simulink model "ScriptDemo"  (R2022b)
settings: configuration reference "TmVcThermal_Configuration_sub" (kept outside this file)
undefined symbols (not defined in the file or in its folder): aaaa, bbbb, cTmComprCtrl_D_u8HvacFlowTable_db, cTmComprCtrl_D_u8HvacFlowTable_sw, cTmComprCtrl_n_i16ChillCmpIMax, cTmComprCtrl_n_i16ChillCmpIMin, cTmComprCtrl_n_i16ChillCmpIMin666, cTmComprCtrl_n_i16ChillCmpPMax, cTmComprCtrl_n_i16ChillCmpPMin, cTmComprCtrl_n_i16CmpChillCoolRpmKiMax, cTmComprCtrl_n_i16CmpChillCoolRpmKiMin, cTmComprCtrl_n_i16CmpChillCoolRpmKpMax, cTmComprCtrl_n_i16CmpChillCoolRpmKpMin, cTmComprCtrl_n_i16CmpCoolRpmKiMax, cTmComprCtrl_n_i16CmpCoolRpmKiMin, cTmComprCtrl_n_i16CmpCoolRpmKpMax, cTmComprCtrl_n_i16CmpCoolRpmKpMin, cTmComprCtrl_n_i16SM4CmpHeatKiMax, cTmComprCtrl_n_i16SM4CmpHeatKiMin, cTmComprCtrl_n_i16SM4CmpHeatKpMax, cTmComprCtrl_n_i16SM4CmpHeatKpMin, cTmComprCtrl_n_i16SM5CmpHeatKiMax, cTmComprCtrl_n_i16SM5CmpHeatKiMin, cTmComprCtrl_n_i16SM5CmpHeatKpMax, cTmComprCtrl_n_i16SM5CmpHeatKpMin, cTmComprCtrl_n_i16SM6CmpHeatKiMax, cTmComprCtrl_n_i16SM6CmpHeatKiMin, cTmComprCtrl_n_i16SM6CmpHeatKpMax, cTmComprCtrl_n_i16SM6CmpHeatKpMin, cTmComprCtrl_n_u16CmpMaxSpdFanFltLimt, cTmComprCtrl_n_u16CmpMaxSpdLoSidePFltLimt, cTmComprCtrl_n_u16CmpMaxSpdSensorFltLimt, cTmComprCtrl_n_u16CompMinRpm, cTmComprCtrl_n_u16CompRpmIncThres, cTmComprCtrl_t_u16BattCooltFFPeriod, cTmComprCtrl_t_u16BattCooltPIPeriod, cTmComprCtrl_t_u16CmpCoolFFPeriod, cTmComprCtrl_t_u16CmpCoolPIPeriod, cTmComprCtrl_t_u16CoolCmpChillFFPeriod, cTmComprCtrl_t_u16CoolCmpChillPIPeriod, cTmComprCtrl_t_u16SM4CmpHeatFFPeriod, cTmComprCtrl_t_u16SM4CmpHeatPIPeriod, cTmComprCtrl_t_u16SM5CmpHeatFFPeriod, cTmComprCtrl_t_u16SM5CmpHeatPIPeriod, cTmComprCtrl_t_u16SM6CmpHeatFFPeriod, cTmComprCtrl_t_u16SM6CmpHeatPIPeriod, cTmComprCtrl_Te_EvapClearInteg, cTmComprCtrl_Te_i16HpReqTempSaturoffset, cTmComprCtrl_Te_i16SatLpReplaceDiff, cTmComprCtrl_Te_i16SM3BatDiffStartEvapDecOffset, cTmComprCtrl_Te_i16SM3EvapLo, cTmComprCtrl_Te_i16SM3TBatDiffEntEvapDecOffset, cTmComprCtrl_Te_i16SM3TBatDiffEntEvapDecOffsetQuit, cTmComprCtrl_Te_s32ErrCmpChillPIContinueCoolH, cTmComprCtrl_Te_s32ErrCmpChillPIContinueCoolL, cTmComprCtrl_Te_s32ErrCmpPIContinueChillH, cTmComprCtrl_Te_s32ErrCmpPIContinueChillL, cTmComprCtrl_Te_s32ErrCmpPIContinueCoolH, cTmComprCtrl_Te_s32ErrCmpPIContinueCoolL, cTmComprCtrl_Te_s32ErrCmpPIContinueHeatH ... (+398)
libraries: simulink x846, PCMULib x711, simulink_need_slupdate x4
(part 14 of 49)

== system ScriptDemo/Change/changeModSizeGcs/Before1/Subsystem3 ==
  rTmComprCtrl_n_u16CompRpmReqModeOut : Inport  OutDataTypeStr=uint16
  sTmDiag_D_u8CmprDischrgTFltSt : Inport  Port=2  OutDataTypeStr=uint8
  sTmDiag_D_u8FanFltSt : Inport  Port=3  OutDataTypeStr=uint8
  sTmDiag_D_u8HiSidePFltSt : Inport  Port=4  OutDataTypeStr=uint8
  sTmDiag_D_u8OutrCondOutTFltSt : Inport  Port=5  OutDataTypeStr=uint8
  sTmIn_n_s32ElacCmprActl : Inport  Port=6  OutDataTypeStr=single
  sTmIn_v_s32VehSpdLgt : Inport  Port=7  OutDataTypeStr=single
  sTmRefriModeMgr_D_u8HpFmCmd : Inport  Port=8  OutDataTypeStr=uint8
  sTmSigProces_Pw_i16ReqPwrForHeat : Inport  Port=9  OutDataTypeStr=int16
  sTmSigProces_Te_s32CompDischarge : Inport  Port=10  OutDataTypeStr=single
  sTmSigProces_md_u16BlwCool : Inport  Port=11  OutDataTypeStr=uint16
  sTmSigProces_p_u16PHighSide : Inport  Port=12  OutDataTypeStr=uint16
  sTmSigProces_p_u16PLowSide : Inport  Port=13  OutDataTypeStr=uint16
  sTmIn_D_u8HeatPump : Inport  Port=14  OutDataTypeStr=uint8
  sTmIn_D_u8ElecDriveline : Inport  Port=15
  sTmSigProces_md_u16BlwHeat : Inport  Port=16  OutDataTypeStr=uint16
  sTmDiag_D_u8LoSidePFltSt : Inport  Port=17  OutDataTypeStr=uint8
  xTmComprCtrl_B_CompOnReqCompOn : Inport  Port=18  OutDataTypeStr=boolean
  rTmComprCtrl_n_u16CompRpmReqFilter : Outport  OutDataTypeStr=uint16
  xTmComprCtrl_B_KeepRpm : Outport  Port=2  OutDataTypeStr=boolean
  xFilter_B_ComprStop : Outport  Port=3  OutDataTypeStr=boolean
  sFilter_n_u16CompMaxRpm : Outport  Port=4  OutDataTypeStr=uint16
  rFilter_p_u16AcHiSideHiCut : Outport  Port=5  OutDataTypeStr=uint16
  rFilter_p_u16CmpLimitNormalP : Outport  Port=6  OutDataTypeStr=uint16
  rFilter_p_u16CmpLimitLowP : Outport  Port=7  OutDataTypeStr=uint16
  rFilter_p_u16CmpLimitMidP : Outport  Port=8  OutDataTypeStr=uint16
  rFilter_p_u16CmpLimitShutDownP : Outport  Port=9  OutDataTypeStr=uint16
  xTmComprCtrl_B_ReduceRpm : Outport  Port=10  OutDataTypeStr=boolean
  wires:
  ? -> [sTmRefriModeMgr_D_u8HPCurMode]
  sTmIn_n_s32ElacCmprActl/1 -> [sTmIn_n_s32ElacCmprActl]
  [rTmComprCtrl_p_u16AcHiSideHiCut] -> rFilter_p_u16AcHiSideHiCut/1
  sTmIn_D_u8HeatPump/1 -> [sTmIn_D_u8HeatPump]
  sTmSigProces_md_u16BlwCool/1 -> [sTmSigProces_md_u16BlwCool]
  sTmDiag_D_u8OutrCondOutTFltSt/1 -> [sTmDiag_D_u8OutrCondOutTFltSt]
  ? -> [sTmSigProces_Te_s32TAmb]
  sTmSigProces_md_u16BlwHeat/1 -> [sTmSigProces_md_u16BlwHeat]
  [rTmComprCtrl_p_u16CmpLimitShutDownP] -> rFilter_p_u16CmpLimitShutDownP/1
  sTmRefriModeMgr_D_u8HpFmCmd/1 -> [sTmRefriModeMgr_D_u8HpFmCmd]
  [rTmComprCtrl_p_u16CmpLimitLowP] -> rFilter_p_u16CmpLimitLowP/1
  sTmDiag_D_u8LoSidePFltSt/1 -> [sTmDiag_D_u8LoSidePFltSt]
  sTmSigProces_p_u16PLowSide/1 -> [sTmSigProces_p_u16PLowSide]
  [rTmComprCtrl_n_u16CompRpmReqCompOn] -> rTmComprCtrl_n_u16CompRpmReqFilter/1
  [xTmComprCtrl_B_ComprStop] -> xFilter_B_ComprStop/1
  sTmIn_D_u8ElecDriveline/1 -> [sTmIn_D_u8ElecDriveline]
  sTmDiag_D_u8HiSidePFltSt/1 -> [sTmDiag_D_u8HiSidePFltSt]
  [sTmComprCtrl_n_u16CompMaxRpm] -> sFilter_n_u16CompMaxRpm/1
  ? -> [sTmSigProces_D_u8CarChrgMode]
  [xTmComprCtrl_B_KeepRpm] -> xTmComprCtrl_B_KeepRpm/1
  sTmDiag_D_u8CmprDischrgTFltSt/1 -> [sTmDiag_D_u8CmprDischrgTFltSt]
  sTmSigProces_p_u16PHighSide/1 -> [sTmSigProces_p_u16PHighSide]
  xTmComprCtrl_B_CompOnReqCompOn/1 -> [xTmComprCtrl_B_CompOnReqCompOn]
  sTmSigProces_Te_s32CompDischarge/1 -> [sTmSigProces_Te_s32CompDischarge]
  [rTmComprCtrl_p_u16CmpLimitMidP] -> rFilter_p_u16CmpLimitMidP/1
  [rTmComprCtrl_p_u16CmpLimitNormalP] -> rFilter_p_u16CmpLimitNormalP/1
  sTmIn_v_s32VehSpdLgt/1 -> [sTmIn_v_s32VehSpdLgt]
  [xTmComprCtrl_B_ReduceRpm] -> xTmComprCtrl_B_ReduceRpm/1
  sTmSigProces_Pw_i16ReqPwrForHeat/1 -> [sTmSigProces_Pw_i16ReqPwrForHeat]
  sTmDiag_D_u8FanFltSt/1 -> [sTmDiag_D_u8FanFltSt]
  rTmComprCtrl_n_u16CompRpmReqModeOut/1 -> [rTmComprCtrl_n_u16CompRpmReqModeOut]

== system ScriptDemo/Create/Model/createModGoto/After ==
  note: % 目的: 为输出端口创建debug 及对应的输入模块
      | [cnt] = createDebug(gcs)
  note: <模型信息: After>
      |
      | 【输入端口】
      | sTmRefriVlvCtrl_X_s32CEXVPosReqIn
      | sTmRefriVlvCtrl_X_s32EEXVPosReqIn
      | sTmRefriVlvCtrl_X_s32BEXVPosReqIn
      | yTmRefriVlvCtrl_B_HpcCexvMovEnableIn
      | sTmRefriVlvCtrl_Z_u8CEXVInitStateIn
      | yTmRefriVlvCtrl_B_CexvCalibReqIn
      | yTmRefriVlvCtrl_B_HpcEexvMovEnableIn
      | sTmRefriVlvCtrl_Z_u8EEXVInitStateIn
      | yTmRefriVlvCtrl_B_EexvCalibReqIn
      | yTmRefriVlvCtrl_B_HpcBexvMovEnableIn
      | sTmRefriVlvCtrl_Z_u8BEXVInitStateIn
      | yTmRefriVlvCtrl_B_BexvCalibReqIn
      | sTmRefriVlvCtrl_X_s32SM3BexvMaxPosIn
      | yTmRefriVlvCtrl_B_EvapBattTLimBexvEnaIn
      | sTmRefriVlvCtrl_D_u8EexvRefriSwitchStIn
      | sTmRefriVlvCtrl_D_u8CexvRefriSwitchStIn
      | sTmRefriVlvCtrl_D_u8BexvRefriSwitchStIn
      |
      | 【输出端口】
      | sTmRefriVlvCtrl_X_s32CEXVPosReq
      | sTmRefriVlvCtrl_X_s32EEXVPosReq
      | sTmRefriVlvCtrl_X_s32BEXVPosReq
      | yTmRefriVlvCtrl_B_HpcCexvMovEnable
      | sTmRefriVlvCtrl_Z_u8CEXVInitState
      | yTmRefriVlvCtrl_B_CexvCalibReq
      | yTmRefriVlvCtrl_B_HpcEexvMovEnable
      | sTmRefriVlvCtrl_Z_u8EEXVInitState
      | yTmRefriVlvCtrl_B_EexvCalibReq
      | yTmRefriVlvCtrl_B_HpcBexvMovEnable
      | sTmRefriVlvCtrl_Z_u8BEXVInitState
      | yTmRefriVlvCtrl_B_BexvCalibReq
      | sTmRefriVlvCtrl_X_s32SM3BexvMaxPos
      | yTmRefriVlvCtrl_B_EvapBattTLimBexvEna
      | sTmRefriVlvCtrl_D_u8EexvRefriSwitchSt
      | sTmRefriVlvCtrl_D_u8CexvRefriSwitchSt
      | sTmRefriVlvCtrl_D_u8BexvRefriSwitchSt
      |
      | 【标定量】
      | 无标定量
      |
      | 创建时间: 2025-03-13 10:33:23
  sTmRefriVlvCtrl_X_s32CEXVPosReqIn : Inport  OutDataTypeStr=single
  sTmRefriVlvCtrl_X_s32EEXVPosReqIn : Inport  Port=2  OutDataTypeStr=single
  sTmRefriVlvCtrl_X_s32BEXVPosReqIn : Inport  Port=3  OutDataTypeStr=single
  yTmRefriVlvCtrl_B_HpcCexvMovEnableIn : Inport  Port=4  OutDataTypeStr=boolean
  sTmRefriVlvCtrl_Z_u8CEXVInitStateIn : Inport  Port=5  OutDataTypeStr=uint8
  yTmRefriVlvCtrl_B_CexvCalibReqIn : Inport  Port=6  OutDataTypeStr=boolean
  yTmRefriVlvCtrl_B_HpcEexvMovEnableIn : Inport  Port=7  OutDataTypeStr=boolean
  sTmRefriVlvCtrl_Z_u8EEXVInitStateIn : Inport  Port=8  OutDataTypeStr=uint8
  yTmRefriVlvCtrl_B_EexvCalibReqIn : Inport  Port=9  OutDataTypeStr=boolean
  yTmRefriVlvCtrl_B_HpcBexvMovEnableIn : Inport  Port=10  OutDataTypeStr=boolean
  sTmRefriVlvCtrl_Z_u8BEXVInitStateIn : Inport  Port=11  OutDataTypeStr=uint8
  yTmRefriVlvCtrl_B_BexvCalibReqIn : Inport  Port=12  OutDataTypeStr=boolean
  sTmRefriVlvCtrl_X_s32SM3BexvMaxPosIn : Inport  Port=13  OutDataTypeStr=single
  yTmRefriVlvCtrl_B_EvapBattTLimBexvEnaIn : Inport  Port=14  OutDataTypeStr=boolean
  sTmRefriVlvCtrl_D_u8EexvRefriSwitchStIn : Inport  Port=15  OutDataTypeStr=uint8
  sTmRefriVlvCtrl_D_u8CexvRefriSwitchStIn : Inport  Port=16  OutDataTypeStr=uint8
  sTmRefriVlvCtrl_D_u8BexvRefriSwitchStIn : Inport  Port=17  OutDataTypeStr=uint8
  OutDebug : PCMULib/Interface/OutdebugRvs  SWI=cTmRefriVlvCtrl_X_s32CEXVPosReq_sw  DBI=cTmRefriVlvCtrl_X_s32CEXVPosReq_db
      settings: SourceProductName=PCMULib
  OutDebug1 : PCMULib/Interface/OutdebugRvs  SWI=cTmRefriVlvCtrl_X_s32EEXVPosReq_sw  DBI=cTmRefriVlvCtrl_X_s32EEXVPosReq_db
      settings: SourceProductName=PCMULib
  OutDebug10 : PCMULib/Interface/OutdebugRvs  SWI=cTmRefriVlvCtrl_Z_u8BEXVInitState_sw  DBI=cTmRefriVlvCtrl_Z_u8BEXVInitState_db
      settings: SourceProductName=PCMULib
  OutDebug11 : PCMULib/Interface/OutdebugRvs  SWI=cTmRefriVlvCtrl_B_BexvCalibReq_sw  DBI=cTmRefriVlvCtrl_B_BexvCalibReq_db
      settings: SourceProductName=PCMULib
  OutDebug12 : PCMULib/Interface/OutdebugRvs  SWI=cTmRefriVlvCtrl_X_s32SM3BexvMaxPos_sw  DBI=cTmRefriVlvCtrl_X_s32SM3BexvMaxPos_db
      settings: SourceProductName=PCMULib
  OutDebug13 : PCMULib/Interface/OutdebugRvs  SWI=cTmRefriVlvCtrl_B_EvapBattTLimBexvEna_sw  DBI=cTmRefriVlvCtrl_B_EvapBattTLimBexvEna_db
      settings: SourceProductName=PCMULib
  OutDebug14 : PCMULib/Interface/OutdebugRvs  SWI=cTmRefriVlvCtrl_D_u8EexvRefriSwitchSt_sw  DBI=cTmRefriVlvCtrl_D_u8EexvRefriSwitchSt_db
      settings: SourceProductName=PCMULib
  OutDebug15 : PCMULib/Interface/OutdebugRvs  SWI=cTmRefriVlvCtrl_D_u8CexvRefriSwitchSt_sw  DBI=cTmRefriVlvCtrl_D_u8CexvRefriSwitchSt_db
      settings: SourceProductName=PCMULib
  OutDebug16 : PCMULib/Interface/OutdebugRvs  SWI=cTmRefriVlvCtrl_D_u8BexvRefriSwitchSt_sw  DBI=cTmRefriVlvCtrl_D_u8BexvRefriSwitchSt_db
      settings: SourceProductName=PCMULib
  OutDebug2 : PCMULib/Interface/OutdebugRvs  SWI=cTmRefriVlvCtrl_X_s32BEXVPosReq_sw  DBI=cTmRefriVlvCtrl_X_s32BEXVPosReq_db
      settings: SourceProductName=PCMULib
  OutDebug3 : PCMULib/Interface/OutdebugRvs  SWI=cTmRefriVlvCtrl_B_HpcCexvMovEnable_sw  DBI=cTmRefriVlvCtrl_B_HpcCexvMovEnable_db
      settings: SourceProductName=PCMULib
  OutDebug4 : PCMULib/Interface/OutdebugRvs  SWI=cTmRefriVlvCtrl_Z_u8CEXVInitState_sw  DBI=cTmRefriVlvCtrl_Z_u8CEXVInitState_db
      settings: SourceProductName=PCMULib
  OutDebug5 : PCMULib/Interface/OutdebugRvs  SWI=cTmRefriVlvCtrl_B_CexvCalibReq_sw  DBI=cTmRefriVlvCtrl_B_CexvCalibReq_db
      settings: SourceProductName=PCMULib
  OutDebug6 : PCMULib/Interface/OutdebugRvs  SWI=cTmRefriVlvCtrl_B_HpcEexvMovEnable_sw  DBI=cTmRefriVlvCtrl_B_HpcEexvMovEnable_db
      settings: SourceProductName=PCMULib
  OutDebug7 : PCMULib/Interface/OutdebugRvs  SWI=cTmRefriVlvCtrl_Z_u8EEXVInitState_sw  DBI=cTmRefriVlvCtrl_Z_u8EEXVInitState_db
      settings: SourceProductName=PCMULib
  OutDebug8 : PCMULib/Interface/OutdebugRvs  SWI=cTmRefriVlvCtrl_B_EexvCalibReq_sw  DBI=cTmRefriVlvCtrl_B_EexvCalibReq_db
      settings: SourceProductName=PCMULib
  OutDebug9 : PCMULib/Interface/OutdebugRvs  SWI=cTmRefriVlvCtrl_B_HpcBexvMovEnable_sw  DBI=cTmRefriVlvCtrl_B_HpcBexvMovEnable_db
      settings: SourceProductName=PCMULib
  sTmRefriVlvCtrl_X_s32CEXVPosReq : Outport  OutDataTypeStr=single
  sTmRefriVlvCtrl_X_s32EEXVPosReq : Outport  Port=2  OutDataTypeStr=single
  sTmRefriVlvCtrl_X_s32BEXVPosReq : Outport  Port=3  OutDataTypeStr=single
  yTmRefriVlvCtrl_B_HpcCexvMovEnable : Outport  Port=4  OutDataTypeStr=boolean
  sTmRefriVlvCtrl_Z_u8CEXVInitState : Outport  Port=5  OutDataTypeStr=uint8
  yTmRefriVlvCtrl_B_CexvCalibReq : Outport  Port=6  OutDataTypeStr=boolean
  yTmRefriVlvCtrl_B_HpcEexvMovEnable : Outport  Port=7  OutDataTypeStr=boolean
  sTmRefriVlvCtrl_Z_u8EEXVInitState : Outport  Port=8  OutDataTypeStr=uint8
  yTmRefriVlvCtrl_B_EexvCalibReq : Outport  Port=9  OutDataTypeStr=boolean
  yTmRefriVlvCtrl_B_HpcBexvMovEnable : Outport  Port=10  OutDataTypeStr=boolean
  sTmRefriVlvCtrl_Z_u8BEXVInitState : Outport  Port=11  OutDataTypeStr=uint8
  yTmRefriVlvCtrl_B_BexvCalibReq : Outport  Port=12  OutDataTypeStr=boolean
  sTmRefriVlvCtrl_X_s32SM3BexvMaxPos : Outport  Port=13  OutDataTypeStr=single
  yTmRefriVlvCtrl_B_EvapBattTLimBexvEna : Outport  Port=14  OutDataTypeStr=boolean
  sTmRefriVlvCtrl_D_u8EexvRefriSwitchSt : Outport  Port=15  OutDataTypeStr=uint8
  sTmRefriVlvCtrl_D_u8CexvRefriSwitchSt : Outport  Port=16  OutDataTypeStr=uint8
  sTmRefriVlvCtrl_D_u8BexvRefriSwitchSt : Outport  Port=17  OutDataTypeStr=uint8
  wires:
  sTmRefriVlvCtrl_X_s32SM3BexvMaxPosIn/1 -> OutDebug12/1
  OutDebug12/1 -> sTmRefriVlvCtrl_X_s32SM3BexvMaxPos/1
  sTmRefriVlvCtrl_X_s32BEXVPosReqIn/1 -> OutDebug2/1
  OutDebug2/1 -> sTmRefriVlvCtrl_X_s32BEXVPosReq/1
  OutDebug16/1 -> sTmRefriVlvCtrl_D_u8BexvRefriSwitchSt/1
  sTmRefriVlvCtrl_D_u8EexvRefriSwitchStIn/1 -> OutDebug14/1
  OutDebug5/1 -> yTmRefriVlvCtrl_B_CexvCalibReq/1
  OutDebug3/1 -> yTmRefriVlvCtrl_B_HpcCexvMovEnable/1
  sTmRefriVlvCtrl_Z_u8CEXVInitStateIn/1 -> OutDebug4/1
  OutDebug4/1 -> sTmRefriVlvCtrl_Z_u8CEXVInitState/1
  sTmRefriVlvCtrl_D_u8BexvRefriSwitchStIn/1 -> OutDebug16/1
  OutDebug1/1 -> sTmRefriVlvCtrl_X_s32EEXVPosReq/1
  OutDebug14/1 -> sTmRefriVlvCtrl_D_u8EexvRefriSwitchSt/1
  yTmRefriVlvCtrl_B_CexvCalibReqIn/1 -> OutDebug5/1
  sTmRefriVlvCtrl_X_s32EEXVPosReqIn/1 -> OutDebug1/1
  yTmRefriVlvCtrl_B_HpcCexvMovEnableIn/1 -> OutDebug3/1
  yTmRefriVlvCtrl_B_EvapBattTLimBexvEnaIn/1 -> OutDebug13/1
  OutDebug13/1 -> yTmRefriVlvCtrl_B_EvapBattTLimBexvEna/1
  sTmRefriVlvCtrl_Z_u8BEXVInitStateIn/1 -> OutDebug10/1
  OutDebug10/1 -> sTmRefriVlvCtrl_Z_u8BEXVInitState/1
  sTmRefriVlvCtrl_D_u8CexvRefriSwitchStIn/1 -> OutDebug15/1
  OutDebug15/1 -> sTmRefriVlvCtrl_D_u8CexvRefriSwitchSt/1
  OutDebug/1 -> sTmRefriVlvCtrl_X_s32CEXVPosReq/1
  OutDebug7/1 -> sTmRefriVlvCtrl_Z_u8EEXVInitState/1
  OutDebug8/1 -> yTmRefriVlvCtrl_B_EexvCalibReq/1
  yTmRefriVlvCtrl_B_EexvCalibReqIn/1 -> OutDebug8/1
  sTmRefriVlvCtrl_X_s32CEXVPosReqIn/1 -> OutDebug/1
  OutDebug6/1 -> yTmRefriVlvCtrl_B_HpcEexvMovEnable/1
  yTmRefriVlvCtrl_B_HpcEexvMovEnableIn/1 -> OutDebug6/1
  sTmRefriVlvCtrl_Z_u8EEXVInitStateIn/1 -> OutDebug7/1
  yTmRefriVlvCtrl_B_HpcBexvMovEnableIn/1 -> OutDebug9/1
  OutDebug9/1 -> yTmRefriVlvCtrl_B_HpcBexvMovEnable/1
  yTmRefriVlvCtrl_B_BexvCalibReqIn/1 -> OutDebug11/1
  OutDebug11/1 -> yTmRefriVlvCtrl_B_BexvCalibReq/1

== system ScriptDemo/Create/Model/createModGoto/After1 ==
  note: % 目的: 为输出端口创建debug 及对应的输入模块
      | [cnt] = createDebug(gcs)
  sTmRefriVlvCtrl_X_s32CEXVPosReqIn : Inport  OutDataTypeStr=single
  sTmRefriVlvCtrl_X_s32EEXVPosReqIn : Inport  Port=2  OutDataTypeStr=single
  sTmRefriVlvCtrl_X_s32BEXVPosReqIn : Inport  Port=3  OutDataTypeStr=single
  yTmRefriVlvCtrl_B_HpcCexvMovEnableIn : Inport  Port=4  OutDataTypeStr=boolean
  sTmRefriVlvCtrl_Z_u8CEXVInitStateIn : Inport  Port=5  OutDataTypeStr=uint8
  yTmRefriVlvCtrl_B_CexvCalibReqIn : Inport  Port=6  OutDataTypeStr=boolean
  yTmRefriVlvCtrl_B_HpcEexvMovEnableIn : Inport  Port=7  OutDataTypeStr=boolean
  sTmRefriVlvCtrl_Z_u8EEXVInitStateIn : Inport  Port=8  OutDataTypeStr=uint8
  yTmRefriVlvCtrl_B_EexvCalibReqIn : Inport  Port=9  OutDataTypeStr=boolean
  yTmRefriVlvCtrl_B_HpcBexvMovEnableIn : Inport  Port=10  OutDataTypeStr=boolean
  sTmRefriVlvCtrl_Z_u8BEXVInitStateIn : Inport  Port=11  OutDataTypeStr=uint8
  yTmRefriVlvCtrl_B_BexvCalibReqIn : Inport  Port=12  OutDataTypeStr=boolean
  sTmRefriVlvCtrl_X_s32SM3BexvMaxPosIn : Inport  Port=13  OutDataTypeStr=single
  yTmRefriVlvCtrl_B_EvapBattTLimBexvEnaIn : Inport  Port=14  OutDataTypeStr=boolean
  sTmRefriVlvCtrl_D_u8EexvRefriSwitchStIn : Inport  Port=15  OutDataTypeStr=uint8
  sTmRefriVlvCtrl_D_u8CexvRefriSwitchStIn : Inport  Port=16  OutDataTypeStr=uint8
  sTmRefriVlvCtrl_D_u8BexvRefriSwitchStIn : Inport  Port=17  OutDataTypeStr=uint8
  OutDebug : PCMULib/Interface/OutdebugRvs  SWI=cTmRefriVlvCtrl_X_s32CEXVPosReq_sw  DBI=cTmRefriVlvCtrl_X_s32CEXVPosReq_db
      settings: SourceProductName=PCMULib
  OutDebug1 : PCMULib/Interface/OutdebugRvs  SWI=cTmRefriVlvCtrl_X_s32EEXVPosReq_sw  DBI=cTmRefriVlvCtrl_X_s32EEXVPosReq_db
      settings: SourceProductName=PCMULib
  OutDebug10 : PCMULib/Interface/OutdebugRvs  SWI=cTmRefriVlvCtrl_Z_u8BEXVInitState_sw  DBI=cTmRefriVlvCtrl_Z_u8BEXVInitState_db
      settings: SourceProductName=PCMULib
  OutDebug11 : PCMULib/Interface/OutdebugRvs  SWI=cTmRefriVlvCtrl_B_BexvCalibReq_sw  DBI=cTmRefriVlvCtrl_B_BexvCalibReq_db
      settings: SourceProductName=PCMULib
  OutDebug12 : PCMULib/Interface/OutdebugRvs  SWI=cTmRefriVlvCtrl_X_s32SM3BexvMaxPos_sw  DBI=cTmRefriVlvCtrl_X_s32SM3BexvMaxPos_db
      settings: SourceProductName=PCMULib
  OutDebug13 : PCMULib/Interface/OutdebugRvs  SWI=cTmRefriVlvCtrl_B_EvapBattTLimBexvEna_sw  DBI=cTmRefriVlvCtrl_B_EvapBattTLimBexvEna_db
      settings: SourceProductName=PCMULib
  OutDebug14 : PCMULib/Interface/OutdebugRvs  SWI=cTmRefriVlvCtrl_D_u8EexvRefriSwitchSt_sw  DBI=cTmRefriVlvCtrl_D_u8EexvRefriSwitchSt_db
      settings: SourceProductName=PCMULib
  OutDebug15 : PCMULib/Interface/OutdebugRvs  SWI=cTmRefriVlvCtrl_D_u8CexvRefriSwitchSt_sw  DBI=cTmRefriVlvCtrl_D_u8CexvRefriSwitchSt_db
      settings: SourceProductName=PCMULib
  OutDebug16 : PCMULib/Interface/OutdebugRvs  SWI=cTmRefriVlvCtrl_D_u8BexvRefriSwitchSt_sw  DBI=cTmRefriVlvCtrl_D_u8BexvRefriSwitchSt_db
      settings: SourceProductName=PCMULib
  OutDebug2 : PCMULib/Interface/OutdebugRvs  SWI=cTmRefriVlvCtrl_X_s32BEXVPosReq_sw  DBI=cTmRefriVlvCtrl_X_s32BEXVPosReq_db
      settings: SourceProductName=PCMULib
  OutDebug3 : PCMULib/Interface/OutdebugRvs  SWI=cTmRefriVlvCtrl_B_HpcCexvMovEnable_sw  DBI=cTmRefriVlvCtrl_B_HpcCexvMovEnable_db
      settings: SourceProductName=PCMULib
  OutDebug4 : PCMULib/Interface/OutdebugRvs  SWI=cTmRefriVlvCtrl_Z_u8CEXVInitState_sw  DBI=cTmRefriVlvCtrl_Z_u8CEXVInitState_db
      settings: SourceProductName=PCMULib
  OutDebug5 : PCMULib/Interface/OutdebugRvs  SWI=cTmRefriVlvCtrl_B_CexvCalibReq_sw  DBI=cTmRefriVlvCtrl_B_CexvCalibReq_db
      settings: SourceProductName=PCMULib
  OutDebug6 : PCMULib/Interface/OutdebugRvs  SWI=cTmRefriVlvCtrl_B_HpcEexvMovEnable_sw  DBI=cTmRefriVlvCtrl_B_HpcEexvMovEnable_db
      settings: SourceProductName=PCMULib
  OutDebug7 : PCMULib/Interface/OutdebugRvs  SWI=cTmRefriVlvCtrl_Z_u8EEXVInitState_sw  DBI=cTmRefriVlvCtrl_Z_u8EEXVInitState_db
      settings: SourceProductName=PCMULib
  OutDebug8 : PCMULib/Interface/OutdebugRvs  SWI=cTmRefriVlvCtrl_B_EexvCalibReq_sw  DBI=cTmRefriVlvCtrl_B_EexvCalibReq_db
      settings: SourceProductName=PCMULib
  OutDebug9 : PCMULib/Interface/OutdebugRvs  SWI=cTmRefriVlvCtrl_B_HpcBexvMovEnable_sw  DBI=cTmRefriVlvCtrl_B_HpcBexvMovEnable_db
      settings: SourceProductName=PCMULib
  sTmRefriVlvCtrl_X_s32CEXVPosReq : Outport  OutDataTypeStr=single
  sTmRefriVlvCtrl_X_s32EEXVPosReq : Outport  Port=2  OutDataTypeStr=single
  sTmRefriVlvCtrl_X_s32BEXVPosReq : Outport  Port=3  OutDataTypeStr=single
  yTmRefriVlvCtrl_B_HpcCexvMovEnable : Outport  Port=4  OutDataTypeStr=boolean
  sTmRefriVlvCtrl_Z_u8CEXVInitState : Outport  Port=5  OutDataTypeStr=uint8
  yTmRefriVlvCtrl_B_CexvCalibReq : Outport  Port=6  OutDataTypeStr=boolean
  yTmRefriVlvCtrl_B_HpcEexvMovEnable : Outport  Port=7  OutDataTypeStr=boolean
  sTmRefriVlvCtrl_Z_u8EEXVInitState : Outport  Port=8  OutDataTypeStr=uint8
  yTmRefriVlvCtrl_B_EexvCalibReq : Outport  Port=9  OutDataTypeStr=boolean
  yTmRefriVlvCtrl_B_HpcBexvMovEnable : Outport  Port=10  OutDataTypeStr=boolean
  sTmRefriVlvCtrl_Z_u8BEXVInitState : Outport  Port=11  OutDataTypeStr=uint8
  yTmRefriVlvCtrl_B_BexvCalibReq : Outport  Port=12  OutDataTypeStr=boolean
  sTmRefriVlvCtrl_X_s32SM3BexvMaxPos : Outport  Port=13  OutDataTypeStr=single
  yTmRefriVlvCtrl_B_EvapBattTLimBexvEna : Outport  Port=14  OutDataTypeStr=boolean
  sTmRefriVlvCtrl_D_u8EexvRefriSwitchSt : Outport  Port=15  OutDataTypeStr=uint8
  sTmRefriVlvCtrl_D_u8CexvRefriSwitchSt : Outport  Port=16  OutDataTypeStr=uint8
  sTmRefriVlvCtrl_D_u8BexvRefriSwitchSt : Outport  Port=17  OutDataTypeStr=uint8
  wires:
  sTmRefriVlvCtrl_X_s32SM3BexvMaxPosIn/1 -> OutDebug12/1
  OutDebug12/1 -> sTmRefriVlvCtrl_X_s32SM3BexvMaxPos/1
  sTmRefriVlvCtrl_X_s32BEXVPosReqIn/1 -> OutDebug2/1
  OutDebug2/1 -> sTmRefriVlvCtrl_X_s32BEXVPosReq/1
  OutDebug16/1 -> sTmRefriVlvCtrl_D_u8BexvRefriSwitchSt/1
  sTmRefriVlvCtrl_D_u8EexvRefriSwitchStIn/1 -> OutDebug14/1
  OutDebug5/1 -> yTmRefriVlvCtrl_B_CexvCalibReq/1
  OutDebug3/1 -> yTmRefriVlvCtrl_B_HpcCexvMovEnable/1
  sTmRefriVlvCtrl_Z_u8CEXVInitStateIn/1 -> OutDebug4/1
  OutDebug4/1 -> sTmRefriVlvCtrl_Z_u8CEXVInitState/1
  sTmRefriVlvCtrl_D_u8BexvRefriSwitchStIn/1 -> OutDebug16/1
  OutDebug1/1 -> sTmRefriVlvCtrl_X_s32EEXVPosReq/1
  OutDebug14/1 -> sTmRefriVlvCtrl_D_u8EexvRefriSwitchSt/1
  yTmRefriVlvCtrl_B_CexvCalibReqIn/1 -> OutDebug5/1
  sTmRefriVlvCtrl_X_s32EEXVPosReqIn/1 -> OutDebug1/1
  yTmRefriVlvCtrl_B_HpcCexvMovEnableIn/1 -> OutDebug3/1
  yTmRefriVlvCtrl_B_EvapBattTLimBexvEnaIn/1 -> OutDebug13/1
  OutDebug13/1 -> yTmRefriVlvCtrl_B_EvapBattTLimBexvEna/1
  sTmRefriVlvCtrl_Z_u8BEXVInitStateIn/1 -> OutDebug10/1
  OutDebug10/1 -> sTmRefriVlvCtrl_Z_u8BEXVInitState/1
  sTmRefriVlvCtrl_D_u8CexvRefriSwitchStIn/1 -> OutDebug15/1
  OutDebug15/1 -> sTmRefriVlvCtrl_D_u8CexvRefriSwitchSt/1
  OutDebug/1 -> sTmRefriVlvCtrl_X_s32CEXVPosReq/1
  OutDebug7/1 -> sTmRefriVlvCtrl_Z_u8EEXVInitState/1
  OutDebug8/1 -> yTmRefriVlvCtrl_B_EexvCalibReq/1
  yTmRefriVlvCtrl_B_EexvCalibReqIn/1 -> OutDebug8/1
  sTmRefriVlvCtrl_X_s32CEXVPosReqIn/1 -> OutDebug/1
  OutDebug6/1 -> yTmRefriVlvCtrl_B_HpcEexvMovEnable/1
  yTmRefriVlvCtrl_B_HpcEexvMovEnableIn/1 -> OutDebug6/1
  sTmRefriVlvCtrl_Z_u8EEXVInitStateIn/1 -> OutDebug7/1
  yTmRefriVlvCtrl_B_HpcBexvMovEnableIn/1 -> OutDebug9/1
  OutDebug9/1 -> yTmRefriVlvCtrl_B_HpcBexvMovEnable/1
  yTmRefriVlvCtrl_B_BexvCalibReqIn/1 -> OutDebug11/1
  OutDebug11/1 -> yTmRefriVlvCtrl_B_BexvCalibReq/1

== system ScriptDemo/Create/Model/createModGoto/After2 ==
  note: % 目的: 为输出端口创建debug 及对应的输入模块
      | [cnt] = createDebug(gcs)
  sTmRefriVlvCtrl_X_s32CEXVPosReqIn : Inport  OutDataTypeStr=single
  sTmRefriVlvCtrl_X_s32EEXVPosReqIn : Inport  Port=2  OutDataTypeStr=single
  sTmRefriVlvCtrl_X_s32BEXVPosReqIn : Inport  Port=3  OutDataTypeStr=single
  yTmRefriVlvCtrl_B_HpcCexvMovEnableIn : Inport  Port=4  OutDataTypeStr=boolean
  sTmRefriVlvCtrl_Z_u8CEXVInitStateIn : Inport  Port=5  OutDataTypeStr=uint8
  yTmRefriVlvCtrl_B_CexvCalibReqIn : Inport  Port=6  OutDataTypeStr=boolean
  yTmRefriVlvCtrl_B_HpcEexvMovEnableIn : Inport  Port=7  OutDataTypeStr=boolean
  sTmRefriVlvCtrl_Z_u8EEXVInitStateIn : Inport  Port=8  OutDataTypeStr=uint8
  yTmRefriVlvCtrl_B_EexvCalibReqIn : Inport  Port=9  OutDataTypeStr=boolean
  yTmRefriVlvCtrl_B_HpcBexvMovEnableIn : Inport  Port=10  OutDataTypeStr=boolean
  sTmRefriVlvCtrl_Z_u8BEXVInitStateIn : Inport  Port=11  OutDataTypeStr=uint8
  yTmRefriVlvCtrl_B_BexvCalibReqIn : Inport  Port=12  OutDataTypeStr=boolean
  sTmRefriVlvCtrl_X_s32SM3BexvMaxPosIn : Inport  Port=13  OutDataTypeStr=single
  yTmRefriVlvCtrl_B_EvapBattTLimBexvEnaIn : Inport  Port=14  OutDataTypeStr=boolean
  sTmRefriVlvCtrl_D_u8EexvRefriSwitchStIn : Inport  Port=15  OutDataTypeStr=uint8
  sTmRefriVlvCtrl_D_u8CexvRefriSwitchStIn : Inport  Port=16  OutDataTypeStr=uint8
  sTmRefriVlvCtrl_D_u8BexvRefriSwitchStIn : Inport  Port=17  OutDataTypeStr=uint8
  OutDebug : PCMULib/Interface/OutdebugRvs  SWI=cTmRefriVlvCtrl_X_s32CEXVPosReq_sw  DBI=cTmRefriVlvCtrl_X_s32CEXVPosReq_db
      settings: SourceProductName=PCMULib
  OutDebug1 : PCMULib/Interface/OutdebugRvs  SWI=cTmRefriVlvCtrl_X_s32EEXVPosReq_sw  DBI=cTmRefriVlvCtrl_X_s32EEXVPosReq_db
      settings: SourceProductName=PCMULib
  OutDebug10 : PCMULib/Interface/OutdebugRvs  SWI=cTmRefriVlvCtrl_Z_u8BEXVInitState_sw  DBI=cTmRefriVlvCtrl_Z_u8BEXVInitState_db
      settings: SourceProductName=PCMULib
  OutDebug11 : PCMULib/Interface/OutdebugRvs  SWI=cTmRefriVlvCtrl_B_BexvCalibReq_sw  DBI=cTmRefriVlvCtrl_B_BexvCalibReq_db
      settings: SourceProductName=PCMULib
  OutDebug12 : PCMULib/Interface/OutdebugRvs  SWI=cTmRefriVlvCtrl_X_s32SM3BexvMaxPos_sw  DBI=cTmRefriVlvCtrl_X_s32SM3BexvMaxPos_db
      settings: SourceProductName=PCMULib
  OutDebug13 : PCMULib/Interface/OutdebugRvs  SWI=cTmRefriVlvCtrl_B_EvapBattTLimBexvEna_sw  DBI=cTmRefriVlvCtrl_B_EvapBattTLimBexvEna_db
      settings: SourceProductName=PCMULib
  OutDebug14 : PCMULib/Interface/OutdebugRvs  SWI=cTmRefriVlvCtrl_D_u8EexvRefriSwitchSt_sw  DBI=cTmRefriVlvCtrl_D_u8EexvRefriSwitchSt_db
      settings: SourceProductName=PCMULib
  OutDebug15 : PCMULib/Interface/OutdebugRvs  SWI=cTmRefriVlvCtrl_D_u8CexvRefriSwitchSt_sw  DBI=cTmRefriVlvCtrl_D_u8CexvRefriSwitchSt_db
      settings: SourceProductName=PCMULib
  OutDebug16 : PCMULib/Interface/OutdebugRvs  SWI=cTmRefriVlvCtrl_D_u8BexvRefriSwitchSt_sw  DBI=cTmRefriVlvCtrl_D_u8BexvRefriSwitchSt_db
      settings: SourceProductName=PCMULib
  OutDebug2 : PCMULib/Interface/OutdebugRvs  SWI=cTmRefriVlvCtrl_X_s32BEXVPosReq_sw  DBI=cTmRefriVlvCtrl_X_s32BEXVPosReq_db
      settings: SourceProductName=PCMULib
  OutDebug3 : PCMULib/Interface/OutdebugRvs  SWI=cTmRefriVlvCtrl_B_HpcCexvMovEnable_sw  DBI=cTmRefriVlvCtrl_B_HpcCexvMovEnable_db
      settings: SourceProductName=PCMULib
  OutDebug4 : PCMULib/Interface/OutdebugRvs  SWI=cTmRefriVlvCtrl_Z_u8CEXVInitState_sw  DBI=cTmRefriVlvCtrl_Z_u8CEXVInitState_db
      settings: SourceProductName=PCMULib
  OutDebug5 : PCMULib/Interface/OutdebugRvs  SWI=cTmRefriVlvCtrl_B_CexvCalibReq_sw  DBI=cTmRefriVlvCtrl_B_CexvCalibReq_db
      settings: SourceProductName=PCMULib
  OutDebug6 : PCMULib/Interface/OutdebugRvs  SWI=cTmRefriVlvCtrl_B_HpcEexvMovEnable_sw  DBI=cTmRefriVlvCtrl_B_HpcEexvMovEnable_db
      settings: SourceProductName=PCMULib
  OutDebug7 : PCMULib/Interface/OutdebugRvs  SWI=cTmRefriVlvCtrl_Z_u8EEXVInitState_sw  DBI=cTmRefriVlvCtrl_Z_u8EEXVInitState_db
      settings: SourceProductName=PCMULib
  OutDebug8 : PCMULib/Interface/OutdebugRvs  SWI=cTmRefriVlvCtrl_B_EexvCalibReq_sw  DBI=cTmRefriVlvCtrl_B_EexvCalibReq_db
      settings: SourceProductName=PCMULib
  OutDebug9 : PCMULib/Interface/OutdebugRvs  SWI=cTmRefriVlvCtrl_B_HpcBexvMovEnable_sw  DBI=cTmRefriVlvCtrl_B_HpcBexvMovEnable_db
      settings: SourceProductName=PCMULib
  sTmRefriVlvCtrl_X_s32CEXVPosReq : Outport  OutDataTypeStr=single
  sTmRefriVlvCtrl_X_s32EEXVPosReq : Outport  Port=2  OutDataTypeStr=single
  sTmRefriVlvCtrl_X_s32BEXVPosReq : Outport  Port=3  OutDataTypeStr=single
  yTmRefriVlvCtrl_B_HpcCexvMovEnable : Outport  Port=4  OutDataTypeStr=boolean
  sTmRefriVlvCtrl_Z_u8CEXVInitState : Outport  Port=5  OutDataTypeStr=uint8
  yTmRefriVlvCtrl_B_CexvCalibReq : Outport  Port=6  OutDataTypeStr=boolean
  yTmRefriVlvCtrl_B_HpcEexvMovEnable : Outport  Port=7  OutDataTypeStr=boolean
  sTmRefriVlvCtrl_Z_u8EEXVInitState : Outport  Port=8  OutDataTypeStr=uint8
  yTmRefriVlvCtrl_B_EexvCalibReq : Outport  Port=9  OutDataTypeStr=boolean
  yTmRefriVlvCtrl_B_HpcBexvMovEnable : Outport  Port=10  OutDataTypeStr=boolean
  sTmRefriVlvCtrl_Z_u8BEXVInitState : Outport  Port=11  OutDataTypeStr=uint8
  yTmRefriVlvCtrl_B_BexvCalibReq : Outport  Port=12  OutDataTypeStr=boolean
  sTmRefriVlvCtrl_X_s32SM3BexvMaxPos : Outport  Port=13  OutDataTypeStr=single
  yTmRefriVlvCtrl_B_EvapBattTLimBexvEna : Outport  Port=14  OutDataTypeStr=boolean
  sTmRefriVlvCtrl_D_u8EexvRefriSwitchSt : Outport  Port=15  OutDataTypeStr=uint8
  sTmRefriVlvCtrl_D_u8CexvRefriSwitchSt : Outport  Port=16  OutDataTypeStr=uint8
  sTmRefriVlvCtrl_D_u8BexvRefriSwitchSt : Outport  Port=17  OutDataTypeStr=uint8
  wires:
  sTmRefriVlvCtrl_X_s32SM3BexvMaxPosIn/1 -> OutDebug12/1
  OutDebug12/1 -> sTmRefriVlvCtrl_X_s32SM3BexvMaxPos/1
  sTmRefriVlvCtrl_X_s32BEXVPosReqIn/1 -> OutDebug2/1
  OutDebug2/1 -> sTmRefriVlvCtrl_X_s32BEXVPosReq/1
  OutDebug16/1 -> sTmRefriVlvCtrl_D_u8BexvRefriSwitchSt/1
  sTmRefriVlvCtrl_D_u8EexvRefriSwitchStIn/1 -> OutDebug14/1
  OutDebug5/1 -> yTmRefriVlvCtrl_B_CexvCalibReq/1
  OutDebug3/1 -> yTmRefriVlvCtrl_B_HpcCexvMovEnable/1
  sTmRefriVlvCtrl_Z_u8CEXVInitStateIn/1 -> OutDebug4/1
  OutDebug4/1 -> sTmRefriVlvCtrl_Z_u8CEXVInitState/1
  sTmRefriVlvCtrl_D_u8BexvRefriSwitchStIn/1 -> OutDebug16/1
  OutDebug1/1 -> sTmRefriVlvCtrl_X_s32EEXVPosReq/1
  OutDebug14/1 -> sTmRefriVlvCtrl_D_u8EexvRefriSwitchSt/1
  yTmRefriVlvCtrl_B_CexvCalibReqIn/1 -> OutDebug5/1
  sTmRefriVlvCtrl_X_s32EEXVPosReqIn/1 -> OutDebug1/1
  yTmRefriVlvCtrl_B_HpcCexvMovEnableIn/1 -> OutDebug3/1
  yTmRefriVlvCtrl_B_EvapBattTLimBexvEnaIn/1 -> OutDebug13/1
  OutDebug13/1 -> yTmRefriVlvCtrl_B_EvapBattTLimBexvEna/1
  sTmRefriVlvCtrl_Z_u8BEXVInitStateIn/1 -> OutDebug10/1
  OutDebug10/1 -> sTmRefriVlvCtrl_Z_u8BEXVInitState/1
  sTmRefriVlvCtrl_D_u8CexvRefriSwitchStIn/1 -> OutDebug15/1
  OutDebug15/1 -> sTmRefriVlvCtrl_D_u8CexvRefriSwitchSt/1
  OutDebug/1 -> sTmRefriVlvCtrl_X_s32CEXVPosReq/1
  OutDebug7/1 -> sTmRefriVlvCtrl_Z_u8EEXVInitState/1
  OutDebug8/1 -> yTmRefriVlvCtrl_B_EexvCalibReq/1
  yTmRefriVlvCtrl_B_EexvCalibReqIn/1 -> OutDebug8/1
  sTmRefriVlvCtrl_X_s32CEXVPosReqIn/1 -> OutDebug/1
  OutDebug6/1 -> yTmRefriVlvCtrl_B_HpcEexvMovEnable/1
  yTmRefriVlvCtrl_B_HpcEexvMovEnableIn/1 -> OutDebug6/1
  sTmRefriVlvCtrl_Z_u8EEXVInitStateIn/1 -> OutDebug7/1
  yTmRefriVlvCtrl_B_HpcBexvMovEnableIn/1 -> OutDebug9/1
  OutDebug9/1 -> yTmRefriVlvCtrl_B_HpcBexvMovEnable/1
  yTmRefriVlvCtrl_B_BexvCalibReqIn/1 -> OutDebug11/1
  OutDebug11/1 -> yTmRefriVlvCtrl_B_BexvCalibReq/1

== system ScriptDemo/Create/Model/createModGoto/After3 ==
  note: % 目的: 为输出端口创建debug 及对应的输入模块
      | [cnt] = createDebug(gcs)
  sTmRefriVlvCtrl_X_s32CEXVPosReqIn : Inport  OutDataTypeStr=single
  sTmRefriVlvCtrl_X_s32EEXVPosReqIn : Inport  Port=2  OutDataTypeStr=single
  sTmRefriVlvCtrl_X_s32BEXVPosReqIn : Inport  Port=3  OutDataTypeStr=single
  yTmRefriVlvCtrl_B_HpcCexvMovEnableIn : Inport  Port=4  OutDataTypeStr=boolean
  sTmRefriVlvCtrl_Z_u8CEXVInitStateIn : Inport  Port=5  OutDataTypeStr=uint8
  yTmRefriVlvCtrl_B_CexvCalibReqIn : Inport  Port=6  OutDataTypeStr=boolean
  yTmRefriVlvCtrl_B_HpcEexvMovEnableIn : Inport  Port=7  OutDataTypeStr=boolean
  sTmRefriVlvCtrl_Z_u8EEXVInitStateIn : Inport  Port=8  OutDataTypeStr=uint8
  yTmRefriVlvCtrl_B_EexvCalibReqIn : Inport  Port=9  OutDataTypeStr=boolean
  yTmRefriVlvCtrl_B_HpcBexvMovEnableIn : Inport  Port=10  OutDataTypeStr=boolean
  sTmRefriVlvCtrl_Z_u8BEXVInitStateIn : Inport  Port=11  OutDataTypeStr=uint8
  yTmRefriVlvCtrl_B_BexvCalibReqIn : Inport  Port=12  OutDataTypeStr=boolean
  sTmRefriVlvCtrl_X_s32SM3BexvMaxPosIn : Inport  Port=13  OutDataTypeStr=single
  yTmRefriVlvCtrl_B_EvapBattTLimBexvEnaIn : Inport  Port=14  OutDataTypeStr=boolean
  sTmRefriVlvCtrl_D_u8EexvRefriSwitchStIn : Inport  Port=15  OutDataTypeStr=uint8
  sTmRefriVlvCtrl_D_u8CexvRefriSwitchStIn : Inport  Port=16  OutDataTypeStr=uint8
  sTmRefriVlvCtrl_D_u8BexvRefriSwitchStIn : Inport  Port=17  OutDataTypeStr=uint8
  OutDebug : PCMULib/Interface/OutdebugRvs  SWI=cTmRefriVlvCtrl_X_s32CEXVPosReq_sw  DBI=cTmRefriVlvCtrl_X_s32CEXVPosReq_db
      settings: SourceProductName=PCMULib
  OutDebug1 : PCMULib/Interface/OutdebugRvs  SWI=cTmRefriVlvCtrl_X_s32EEXVPosReq_sw  DBI=cTmRefriVlvCtrl_X_s32EEXVPosReq_db
      settings: SourceProductName=PCMULib
  OutDebug10 : PCMULib/Interface/OutdebugRvs  SWI=cTmRefriVlvCtrl_Z_u8BEXVInitState_sw  DBI=cTmRefriVlvCtrl_Z_u8BEXVInitState_db
      settings: SourceProductName=PCMULib
  OutDebug11 : PCMULib/Interface/OutdebugRvs  SWI=cTmRefriVlvCtrl_B_BexvCalibReq_sw  DBI=cTmRefriVlvCtrl_B_BexvCalibReq_db
      settings: SourceProductName=PCMULib
  OutDebug12 : PCMULib/Interface/OutdebugRvs  SWI=cTmRefriVlvCtrl_X_s32SM3BexvMaxPos_sw  DBI=cTmRefriVlvCtrl_X_s32SM3BexvMaxPos_db
      settings: SourceProductName=PCMULib
  OutDebug13 : PCMULib/Interface/OutdebugRvs  SWI=cTmRefriVlvCtrl_B_EvapBattTLimBexvEna_sw  DBI=cTmRefriVlvCtrl_B_EvapBattTLimBexvEna_db
      settings: SourceProductName=PCMULib
  OutDebug14 : PCMULib/Interface/OutdebugRvs  SWI=cTmRefriVlvCtrl_D_u8EexvRefriSwitchSt_sw  DBI=cTmRefriVlvCtrl_D_u8EexvRefriSwitchSt_db
      settings: SourceProductName=PCMULib
  OutDebug15 : PCMULib/Interface/OutdebugRvs  SWI=cTmRefriVlvCtrl_D_u8CexvRefriSwitchSt_sw  DBI=cTmRefriVlvCtrl_D_u8CexvRefriSwitchSt_db
      settings: SourceProductName=PCMULib
  OutDebug16 : PCMULib/Interface/OutdebugRvs  SWI=cTmRefriVlvCtrl_D_u8BexvRefriSwitchSt_sw  DBI=cTmRefriVlvCtrl_D_u8BexvRefriSwitchSt_db
      settings: SourceProductName=PCMULib
  OutDebug2 : PCMULib/Interface/OutdebugRvs  SWI=cTmRefriVlvCtrl_X_s32BEXVPosReq_sw  DBI=cTmRefriVlvCtrl_X_s32BEXVPosReq_db
      settings: SourceProductName=PCMULib
  OutDebug3 : PCMULib/Interface/OutdebugRvs  SWI=cTmRefriVlvCtrl_B_HpcCexvMovEnable_sw  DBI=cTmRefriVlvCtrl_B_HpcCexvMovEnable_db
      settings: SourceProductName=PCMULib
  OutDebug4 : PCMULib/Interface/OutdebugRvs  SWI=cTmRefriVlvCtrl_Z_u8CEXVInitState_sw  DBI=cTmRefriVlvCtrl_Z_u8CEXVInitState_db
      settings: SourceProductName=PCMULib
  OutDebug5 : PCMULib/Interface/OutdebugRvs  SWI=cTmRefriVlvCtrl_B_CexvCalibReq_sw  DBI=cTmRefriVlvCtrl_B_CexvCalibReq_db
      settings: SourceProductName=PCMULib
  OutDebug6 : PCMULib/Interface/OutdebugRvs  SWI=cTmRefriVlvCtrl_B_HpcEexvMovEnable_sw  DBI=cTmRefriVlvCtrl_B_HpcEexvMovEnable_db
      settings: SourceProductName=PCMULib
  OutDebug7 : PCMULib/Interface/OutdebugRvs  SWI=cTmRefriVlvCtrl_Z_u8EEXVInitState_sw  DBI=cTmRefriVlvCtrl_Z_u8EEXVInitState_db
      settings: SourceProductName=PCMULib
  OutDebug8 : PCMULib/Interface/OutdebugRvs  SWI=cTmRefriVlvCtrl_B_EexvCalibReq_sw  DBI=cTmRefriVlvCtrl_B_EexvCalibReq_db
      settings: SourceProductName=PCMULib
  OutDebug9 : PCMULib/Interface/OutdebugRvs  SWI=cTmRefriVlvCtrl_B_HpcBexvMovEnable_sw  DBI=cTmRefriVlvCtrl_B_HpcBexvMovEnable_db
      settings: SourceProductName=PCMULib
  sTmRefriVlvCtrl_X_s32CEXVPosReq : Outport  OutDataTypeStr=single
  sTmRefriVlvCtrl_X_s32EEXVPosReq : Outport  Port=2  OutDataTypeStr=single
  sTmRefriVlvCtrl_X_s32BEXVPosReq : Outport  Port=3  OutDataTypeStr=single
  yTmRefriVlvCtrl_B_HpcCexvMovEnable : Outport  Port=4  OutDataTypeStr=boolean
  sTmRefriVlvCtrl_Z_u8CEXVInitState : Outport  Port=5  OutDataTypeStr=uint8
  yTmRefriVlvCtrl_B_CexvCalibReq : Outport  Port=6  OutDataTypeStr=boolean
  yTmRefriVlvCtrl_B_HpcEexvMovEnable : Outport  Port=7  OutDataTypeStr=boolean
  sTmRefriVlvCtrl_Z_u8EEXVInitState : Outport  Port=8  OutDataTypeStr=uint8
  yTmRefriVlvCtrl_B_EexvCalibReq : Outport  Port=9  OutDataTypeStr=boolean
  yTmRefriVlvCtrl_B_HpcBexvMovEnable : Outport  Port=10  OutDataTypeStr=boolean
  sTmRefriVlvCtrl_Z_u8BEXVInitState : Outport  Port=11  OutDataTypeStr=uint8
  yTmRefriVlvCtrl_B_BexvCalibReq : Outport  Port=12  OutDataTypeStr=boolean
  sTmRefriVlvCtrl_X_s32SM3BexvMaxPos : Outport  Port=13  OutDataTypeStr=single
  yTmRefriVlvCtrl_B_EvapBattTLimBexvEna : Outport  Port=14  OutDataTypeStr=boolean
  sTmRefriVlvCtrl_D_u8EexvRefriSwitchSt : Outport  Port=15  OutDataTypeStr=uint8
  sTmRefriVlvCtrl_D_u8CexvRefriSwitchSt : Outport  Port=16  OutDataTypeStr=uint8
  sTmRefriVlvCtrl_D_u8BexvRefriSwitchSt : Outport  Port=17  OutDataTypeStr=uint8
  wires:
  sTmRefriVlvCtrl_X_s32SM3BexvMaxPosIn/1 -> OutDebug12/1
  OutDebug12/1 -> sTmRefriVlvCtrl_X_s32SM3BexvMaxPos/1
  sTmRefriVlvCtrl_X_s32BEXVPosReqIn/1 -> OutDebug2/1
  OutDebug2/1 -> sTmRefriVlvCtrl_X_s32BEXVPosReq/1
  OutDebug16/1 -> sTmRefriVlvCtrl_D_u8BexvRefriSwitchSt/1
  sTmRefriVlvCtrl_D_u8EexvRefriSwitchStIn/1 -> OutDebug14/1
  OutDebug5/1 -> yTmRefriVlvCtrl_B_CexvCalibReq/1
  OutDebug3/1 -> yTmRefriVlvCtrl_B_HpcCexvMovEnable/1
  sTmRefriVlvCtrl_Z_u8CEXVInitStateIn/1 -> OutDebug4/1
  OutDebug4/1 -> sTmRefriVlvCtrl_Z_u8CEXVInitState/1
  sTmRefriVlvCtrl_D_u8BexvRefriSwitchStIn/1 -> OutDebug16/1
  OutDebug1/1 -> sTmRefriVlvCtrl_X_s32EEXVPosReq/1
  OutDebug14/1 -> sTmRefriVlvCtrl_D_u8EexvRefriSwitchSt/1
  yTmRefriVlvCtrl_B_CexvCalibReqIn/1 -> OutDebug5/1
  sTmRefriVlvCtrl_X_s32EEXVPosReqIn/1 -> OutDebug1/1
  yTmRefriVlvCtrl_B_HpcCexvMovEnableIn/1 -> OutDebug3/1
  yTmRefriVlvCtrl_B_EvapBattTLimBexvEnaIn/1 -> OutDebug13/1
  OutDebug13/1 -> yTmRefriVlvCtrl_B_EvapBattTLimBexvEna/1
  sTmRefriVlvCtrl_Z_u8BEXVInitStateIn/1 -> OutDebug10/1
  OutDebug10/1 -> sTmRefriVlvCtrl_Z_u8BEXVInitState/1
  sTmRefriVlvCtrl_D_u8CexvRefriSwitchStIn/1 -> OutDebug15/1
  OutDebug15/1 -> sTmRefriVlvCtrl_D_u8CexvRefriSwitchSt/1
  OutDebug/1 -> sTmRefriVlvCtrl_X_s32CEXVPosReq/1
  OutDebug7/1 -> sTmRefriVlvCtrl_Z_u8EEXVInitState/1
  OutDebug8/1 -> yTmRefriVlvCtrl_B_EexvCalibReq/1
  yTmRefriVlvCtrl_B_EexvCalibReqIn/1 -> OutDebug8/1
  sTmRefriVlvCtrl_X_s32CEXVPosReqIn/1 -> OutDebug/1
  OutDebug6/1 -> yTmRefriVlvCtrl_B_HpcEexvMovEnable/1
  yTmRefriVlvCtrl_B_HpcEexvMovEnableIn/1 -> OutDebug6/1
  sTmRefriVlvCtrl_Z_u8EEXVInitStateIn/1 -> OutDebug7/1
  yTmRefriVlvCtrl_B_HpcBexvMovEnableIn/1 -> OutDebug9/1
  OutDebug9/1 -> yTmRefriVlvCtrl_B_HpcBexvMovEnable/1
  yTmRefriVlvCtrl_B_BexvCalibReqIn/1 -> OutDebug11/1
  OutDebug11/1 -> yTmRefriVlvCtrl_B_BexvCalibReq/1

== system ScriptDemo/Create/Model/createModGoto/Before ==
  note: % 目的: 为输出端口创建debug 及对应的输入模块
      | [cnt] = createDebug(gcs)
  note: <模型信息: Before>
      |
      |
      | 【输入端口】
      | sTmRefriVlvCtrl_X_s32CEXVPosReqIn
      | sTmRefriVlvCtrl_X_s32EEXVPosReqIn
      | sTmRefriVlvCtrl_X_s32BEXVPosReqIn
      | yTmRefriVlvCtrl_B_HpcCexvMovEnableIn
      | sTmRefriVlvCtrl_Z_u8CEXVInitStateIn
      | yTmRefriVlvCtrl_B_CexvCalibReqIn
      | yTmRefriVlvCtrl_B_HpcEexvMovEnableIn
      | sTmRefriVlvCtrl_Z_u8EEXVInitStateIn
      | yTmRefriVlvCtrl_B_EexvCalibReqIn
      | yTmRefriVlvCtrl_B_HpcBexvMovEnableIn
      | sTmRefriVlvCtrl_Z_u8BEXVInitStateIn
      | yTmRefriVlvCtrl_B_BexvCalibReqIn
      | sTmRefriVlvCtrl_X_s32SM3BexvMaxPosIn
      | yTmRefriVlvCtrl_B_EvapBattTLimBexvEnaIn
      | sTmRefriVlvCtrl_D_u8EexvRefriSwitchStIn
      | sTmRefriVlvCtrl_D_u8CexvRefriSwitchStIn
      | sTmRefriVlvCtrl_D_u8BexvRefriSwitchStIn
      |
      | 【输出端口】
      | sTmRefriVlvCtrl_X_s32CEXVPosReq
      | sTmRefriVlvCtrl_X_s32EEXVPosReq
      | sTmRefriVlvCtrl_X_s32BEXVPosReq
      | yTmRefriVlvCtrl_B_HpcCexvMovEnable
      | sTmRefriVlvCtrl_Z_u8CEXVInitState
      | yTmRefriVlvCtrl_B_CexvCalibReq
      | yTmRefriVlvCtrl_B_HpcEexvMovEnable
      | sTmRefriVlvCtrl_Z_u8EEXVInitState
      | yTmRefriVlvCtrl_B_EexvCalibReq
      | yTmRefriVlvCtrl_B_HpcBexvMovEnable
      | sTmRefriVlvCtrl_Z_u8BEXVInitState
      | yTmRefriVlvCtrl_B_BexvCalibReq
      | sTmRefriVlvCtrl_X_s32SM3BexvMaxPos
      | yTmRefriVlvCtrl_B_EvapBattTLimBexvEna
      | sTmRefriVlvCtrl_D_u8EexvRefriSwitchSt
      | sTmRefriVlvCtrl_D_u8CexvRefriSwitchSt
      | sTmRefriVlvCtrl_D_u8BexvRefriSwitchSt
      |
      | 【标定量】
      | cTmRefriVlvCtrl_B_BexvCalibReq_db=0
      | cTmRefriVlvCtrl_B_BexvCalibReq_sw=0
      | cTmRefriVlvCtrl_B_CexvCalibReq_db=0
      | cTmRefriVlvCtrl_B_CexvCalibReq_sw=0
      | cTmRefriVlvCtrl_B_EexvCalibReq_db=0
      | cTmRefriVlvCtrl_B_EexvCalibReq_sw=0
      | cTmRefriVlvCtrl_B_EvapBattTLimBexvEna_db=0
      | cTmRefriVlvCtrl_B_EvapBattTLimBexvEna_sw=0
      | cTmRefriVlvCtrl_B_HpcBexvMovEnable_db=0
      | cTmRefriVlvCtrl_B_HpcBexvMovEnable_sw=0
      | cTmRefriVlvCtrl_B_HpcCexvMovEnable_db=0
      | cTmRefriVlvCtrl_B_HpcCexvMovEnable_sw=0
      | cTmRefriVlvCtrl_B_HpcEexvMovEnable_db=0
      | cTmRefriVlvCtrl_B_HpcEexvMovEnable_sw=0
      | cTmRefriVlvCtrl_D_u8BexvRefriSwitchSt_db=0
      | cTmRefriVlvCtrl_D_u8BexvRefriSwitchSt_sw=0
      | cTmRefriVlvCtrl_D_u8CexvRefriSwitchSt_db=0
      | cTmRefriVlvCtrl_D_u8CexvRefriSwitchSt_sw=0
      | cTmRefriVlvCtrl_D_u8EexvRefriSwitchSt_db=0
      | cTmRefriVlvCtrl_D_u8EexvRefriSwitchSt_sw=0
      | cTmRefriVlvCtrl_X_s32BEXVPosReq_db=0
      | cTmRefriVlvCtrl_X_s32BEXVPosReq_sw=0
      | cTmRefriVlvCtrl_X_s32CEXVPosReq_db=0
      | cTmRefriVlvCtrl_X_s32CEXVPosReq_sw=0
      | cTmRefriVlvCtrl_X_s32EEXVPosReq_db=0
      | cTmRefriVlvCtrl_X_s32EEXVPosReq_sw=0
      | cTmRefriVlvCtrl_X_s32SM3BexvMaxPos_db=0
      | cTmRefriVlvCtrl_X_s32SM3BexvMaxPos_sw=0
      | cTmRefriVlvCtrl_Z_u8BEXVInitState_db=0
      | cTmRefriVlvCtrl_Z_u8BEXVInitState_sw=0
      | cTmRefriVlvCtrl_Z_u8CEXVInitState_db=0
      | cTmRefriVlvCtrl_Z_u8CEXVInitState_sw=0
      | cTmRefriVlvCtrl_Z_u8EEXVInitState_db=0
      | cTmRefriVlvCtrl_Z_u8EEXVInitState_sw=0
      |
      | 创建时间: 2025-04-28 16:54:19
  sTmRefriVlvCtrl_X_s32CEXVPosReqIn : Inport  OutDataTypeStr=single
  sTmRefriVlvCtrl_X_s32EEXVPosReqIn : Inport  Port=2  OutDataTypeStr=single
  sTmRefriVlvCtrl_X_s32BEXVPosReqIn : Inport  Port=3  OutDataTypeStr=single
  yTmRefriVlvCtrl_B_HpcCexvMovEnableIn : Inport  Port=4  OutDataTypeStr=boolean
  sTmRefriVlvCtrl_Z_u8CEXVInitStateIn : Inport  Port=5  OutDataTypeStr=uint8
  yTmRefriVlvCtrl_B_CexvCalibReqIn : Inport  Port=6  OutDataTypeStr=boolean
  yTmRefriVlvCtrl_B_HpcEexvMovEnableIn : Inport  Port=7  OutDataTypeStr=boolean
  sTmRefriVlvCtrl_Z_u8EEXVInitStateIn : Inport  Port=8  OutDataTypeStr=uint8
  yTmRefriVlvCtrl_B_EexvCalibReqIn : Inport  Port=9  OutDataTypeStr=boolean
  yTmRefriVlvCtrl_B_HpcBexvMovEnableIn : Inport  Port=10  OutDataTypeStr=boolean
  sTmRefriVlvCtrl_Z_u8BEXVInitStateIn : Inport  Port=11  OutDataTypeStr=uint8
  yTmRefriVlvCtrl_B_BexvCalibReqIn : Inport  Port=12  OutDataTypeStr=boolean
  sTmRefriVlvCtrl_X_s32SM3BexvMaxPosIn : Inport  Port=13  OutDataTypeStr=single
  yTmRefriVlvCtrl_B_EvapBattTLimBexvEnaIn : Inport  Port=14  OutDataTypeStr=boolean
  sTmRefriVlvCtrl_D_u8EexvRefriSwitchStIn : Inport  Port=15  OutDataTypeStr=uint8
  sTmRefriVlvCtrl_D_u8CexvRefriSwitchStIn : Inport  Port=16  OutDataTypeStr=uint8
  sTmRefriVlvCtrl_D_u8BexvRefriSwitchStIn : Inport  Port=17  OutDataTypeStr=uint8
  OutDebug : PCMULib/Interface/OutdebugRvs  SWI=cTmRefriVlvCtrl_X_s32CEXVPosReq_sw  DBI=cTmRefriVlvCtrl_X_s32CEXVPosReq_db
      settings: SourceProductName=PCMULib
  OutDebug1 : PCMULib/Interface/OutdebugRvs  SWI=cTmRefriVlvCtrl_X_s32EEXVPosReq_sw  DBI=cTmRefriVlvCtrl_X_s32EEXVPosReq_db
      settings: SourceProductName=PCMULib
  OutDebug10 : PCMULib/Interface/OutdebugRvs  SWI=cTmRefriVlvCtrl_Z_u8BEXVInitState_sw  DBI=cTmRefriVlvCtrl_Z_u8BEXVInitState_db
      settings: SourceProductName=PCMULib
  OutDebug11 : PCMULib/Interface/OutdebugRvs  SWI=cTmRefriVlvCtrl_B_BexvCalibReq_sw  DBI=cTmRefriVlvCtrl_B_BexvCalibReq_db
      settings: SourceProductName=PCMULib
  OutDebug12 : PCMULib/Interface/OutdebugRvs  SWI=cTmRefriVlvCtrl_X_s32SM3BexvMaxPos_sw  DBI=cTmRefriVlvCtrl_X_s32SM3BexvMaxPos_db
      settings: SourceProductName=PCMULib
  OutDebug13 : PCMULib/Interface/OutdebugRvs  SWI=cTmRefriVlvCtrl_B_EvapBattTLimBexvEna_sw  DBI=cTmRefriVlvCtrl_B_EvapBattTLimBexvEna_db
      settings: SourceProductName=PCMULib
  OutDebug14 : PCMULib/Interface/OutdebugRvs  SWI=cTmRefriVlvCtrl_D_u8EexvRefriSwitchSt_sw  DBI=cTmRefriVlvCtrl_D_u8EexvRefriSwitchSt_db
      settings: SourceProductName=PCMULib
  OutDebug15 : PCMULib/Interface/OutdebugRvs  SWI=cTmRefriVlvCtrl_D_u8CexvRefriSwitchSt_sw  DBI=cTmRefriVlvCtrl_D_u8CexvRefriSwitchSt_db
      settings: SourceProductName=PCMULib
  OutDebug16 : PCMULib/Interface/OutdebugRvs  SWI=cTmRefriVlvCtrl_D_u8BexvRefriSwitchSt_sw  DBI=cTmRefriVlvCtrl_D_u8BexvRefriSwitchSt_db
      settings: SourceProductName=PCMULib
  OutDebug2 : PCMULib/Interface/OutdebugRvs  SWI=cTmRefriVlvCtrl_X_s32BEXVPosReq_sw  DBI=cTmRefriVlvCtrl_X_s32BEXVPosReq_db
      settings: SourceProductName=PCMULib
  OutDebug3 : PCMULib/Interface/OutdebugRvs  SWI=cTmRefriVlvCtrl_B_HpcCexvMovEnable_sw  DBI=cTmRefriVlvCtrl_B_HpcCexvMovEnable_db
      settings: SourceProductName=PCMULib
  OutDebug4 : PCMULib/Interface/OutdebugRvs  SWI=cTmRefriVlvCtrl_Z_u8CEXVInitState_sw  DBI=cTmRefriVlvCtrl_Z_u8CEXVInitState_db
      settings: SourceProductName=PCMULib
  OutDebug5 : PCMULib/Interface/OutdebugRvs  SWI=cTmRefriVlvCtrl_B_CexvCalibReq_sw  DBI=cTmRefriVlvCtrl_B_CexvCalibReq_db
      settings: SourceProductName=PCMULib
  OutDebug6 : PCMULib/Interface/OutdebugRvs  SWI=cTmRefriVlvCtrl_B_HpcEexvMovEnable_sw  DBI=cTmRefriVlvCtrl_B_HpcEexvMovEnable_db
      settings: SourceProductName=PCMULib
  OutDebug7 : PCMULib/Interface/OutdebugRvs  SWI=cTmRefriVlvCtrl_Z_u8EEXVInitState_sw  DBI=cTmRefriVlvCtrl_Z_u8EEXVInitState_db
      settings: SourceProductName=PCMULib
  OutDebug8 : PCMULib/Interface/OutdebugRvs  SWI=cTmRefriVlvCtrl_B_EexvCalibReq_sw  DBI=cTmRefriVlvCtrl_B_EexvCalibReq_db
      settings: SourceProductName=PCMULib
  OutDebug9 : PCMULib/Interface/OutdebugRvs  SWI=cTmRefriVlvCtrl_B_HpcBexvMovEnable_sw  DBI=cTmRefriVlvCtrl_B_HpcBexvMovEnable_db
      settings: SourceProductName=PCMULib
  sTmRefriVlvCtrl_X_s32CEXVPosReq : Outport  OutDataTypeStr=single
  sTmRefriVlvCtrl_X_s32EEXVPosReq : Outport  Port=2  OutDataTypeStr=single
  sTmRefriVlvCtrl_X_s32BEXVPosReq : Outport  Port=3  OutDataTypeStr=single
  yTmRefriVlvCtrl_B_HpcCexvMovEnable : Outport  Port=4  OutDataTypeStr=boolean
  sTmRefriVlvCtrl_Z_u8CEXVInitState : Outport  Port=5  OutDataTypeStr=uint8
  yTmRefriVlvCtrl_B_CexvCalibReq : Outport  Port=6  OutDataTypeStr=boolean
  yTmRefriVlvCtrl_B_HpcEexvMovEnable : Outport  Port=7  OutDataTypeStr=boolean
  sTmRefriVlvCtrl_Z_u8EEXVInitState : Outport  Port=8  OutDataTypeStr=uint8
  yTmRefriVlvCtrl_B_EexvCalibReq : Outport  Port=9  OutDataTypeStr=boolean
  yTmRefriVlvCtrl_B_HpcBexvMovEnable : Outport  Port=10  OutDataTypeStr=boolean
  sTmRefriVlvCtrl_Z_u8BEXVInitState : Outport  Port=11  OutDataTypeStr=uint8
  yTmRefriVlvCtrl_B_BexvCalibReq : Outport  Port=12  OutDataTypeStr=boolean
  sTmRefriVlvCtrl_X_s32SM3BexvMaxPos : Outport  Port=13  OutDataTypeStr=single
  yTmRefriVlvCtrl_B_EvapBattTLimBexvEna : Outport  Port=14  OutDataTypeStr=boolean
  sTmRefriVlvCtrl_D_u8EexvRefriSwitchSt : Outport  Port=15  OutDataTypeStr=uint8
  sTmRefriVlvCtrl_D_u8CexvRefriSwitchSt : Outport  Port=16  OutDataTypeStr=uint8
  sTmRefriVlvCtrl_D_u8BexvRefriSwitchSt : Outport  Port=17  OutDataTypeStr=uint8
  wires:
  sTmRefriVlvCtrl_X_s32SM3BexvMaxPosIn/1 -> OutDebug12/1
  OutDebug12/1 -> sTmRefriVlvCtrl_X_s32SM3BexvMaxPos/1
  sTmRefriVlvCtrl_X_s32BEXVPosReqIn/1 -> OutDebug2/1
  OutDebug2/1 -> sTmRefriVlvCtrl_X_s32BEXVPosReq/1
  OutDebug16/1 -> sTmRefriVlvCtrl_D_u8BexvRefriSwitchSt/1
  sTmRefriVlvCtrl_D_u8EexvRefriSwitchStIn/1 -> OutDebug14/1
  OutDebug5/1 -> yTmRefriVlvCtrl_B_CexvCalibReq/1
  OutDebug3/1 -> yTmRefriVlvCtrl_B_HpcCexvMovEnable/1
  sTmRefriVlvCtrl_Z_u8CEXVInitStateIn/1 -> OutDebug4/1
  OutDebug4/1 -> sTmRefriVlvCtrl_Z_u8CEXVInitState/1
  sTmRefriVlvCtrl_D_u8BexvRefriSwitchStIn/1 -> OutDebug16/1
  OutDebug1/1 -> sTmRefriVlvCtrl_X_s32EEXVPosReq/1
  OutDebug14/1 -> sTmRefriVlvCtrl_D_u8EexvRefriSwitchSt/1
  yTmRefriVlvCtrl_B_CexvCalibReqIn/1 -> OutDebug5/1
  sTmRefriVlvCtrl_X_s32EEXVPosReqIn/1 -> OutDebug1/1
  yTmRefriVlvCtrl_B_HpcCexvMovEnableIn/1 -> OutDebug3/1
  yTmRefriVlvCtrl_B_EvapBattTLimBexvEnaIn/1 -> OutDebug13/1
  OutDebug13/1 -> yTmRefriVlvCtrl_B_EvapBattTLimBexvEna/1
  sTmRefriVlvCtrl_Z_u8BEXVInitStateIn/1 -> OutDebug10/1
  OutDebug10/1 -> sTmRefriVlvCtrl_Z_u8BEXVInitState/1
  sTmRefriVlvCtrl_D_u8CexvRefriSwitchStIn/1 -> OutDebug15/1
  OutDebug15/1 -> sTmRefriVlvCtrl_D_u8CexvRefriSwitchSt/1
  OutDebug/1 -> sTmRefriVlvCtrl_X_s32CEXVPosReq/1
  OutDebug7/1 -> sTmRefriVlvCtrl_Z_u8EEXVInitState/1
  OutDebug8/1 -> yTmRefriVlvCtrl_B_EexvCalibReq/1
  yTmRefriVlvCtrl_B_EexvCalibReqIn/1 -> OutDebug8/1
  sTmRefriVlvCtrl_X_s32CEXVPosReqIn/1 -> OutDebug/1
  OutDebug6/1 -> yTmRefriVlvCtrl_B_HpcEexvMovEnable/1
  yTmRefriVlvCtrl_B_HpcEexvMovEnableIn/1 -> OutDebug6/1
  sTmRefriVlvCtrl_Z_u8EEXVInitStateIn/1 -> OutDebug7/1
  yTmRefriVlvCtrl_B_HpcBexvMovEnableIn/1 -> OutDebug9/1
  OutDebug9/1 -> yTmRefriVlvCtrl_B_HpcBexvMovEnable/1
  yTmRefriVlvCtrl_B_BexvCalibReqIn/1 -> OutDebug11/1
  OutDebug11/1 -> yTmRefriVlvCtrl_B_BexvCalibReq/1

== system ScriptDemo/Create/Model/createModGotoAll/After ==
  note: createModGotoAll()
      |
      | # 在此路径下执行
  AFFaultLimit : Subsystem
  LoSidePFltLimt : Subsystem
  SensFaultLimit : Subsystem
  TAmbLimit : Subsystem
  wires:
  [sTmDiag_D_u8FanFltSt] -> AFFaultLimit/1(sTmDiag_D_u8FanFltSt)
  AFFaultLimit/1(rTmComprCtrl_n_u16CompMaxRpmAfFlt) -> [rTmComprCtrl_n_u16CompMaxRpmAfFlt]
  AFFaultLimit/2(xTmComprCtrl_B_CmpFanFltLimtFlag) -> [xTmComprCtrl_B_CmpFanFltLimtFlag]
  [sTmDiag_D_u8LoSidePFltSt] -> LoSidePFltLimt/1(sTmDiag_D_u8LoSidePFltSt)
  [sTmSigProces_Te_s32TAmb] -> ?
  [sTmIn_D_u8HeatPump] -> LoSidePFltLimt/2(sTmIn_D_u8HeatPump)
  LoSidePFltLimt/1(rTmComprCtrl_n_u16CompMaxRpmLoSidePFlt) -> [rTmComprCtrl_n_u16CompMaxRpmLoSidePFlt]
  LoSidePFltLimt/2(xTmComprCtrl_B_CmpLoSidePFltLimtFlag) -> [xTmComprCtrl_B_CmpLoSidePFltLimtFlag]
  [sTmDiag_D_u8CmprDischrgTFltSt] -> SensFaultLimit/1(sTmDiag_D_u8CmprDischrgTFltSt)
  [sTmDiag_D_u8HiSidePFltSt] -> SensFaultLimit/2(sTmDiag_D_u8HiSidePFltSt)
  [sTmDiag_D_u8OutrCondOutTFltSt] -> SensFaultLimit/3(sTmDiag_D_u8OutrCondOutTFltSt)
  [sTmIn_D_u8HeatPump] -> SensFaultLimit/4(sTmIn_D_u8HeatPump)
  [sTmDiag_D_u8HiSidePNHPFltSt] -> SensFaultLimit/5(sTmDiag_D_u8HiSidePNHPFltSt)
  SensFaultLimit/1(rTmComprCtrl_n_u16CompMaxRpmSensFlt) -> [rTmComprCtrl_n_u16CompMaxRpmSensFlt]
  SensFaultLimit/2(xTmComprCtrl_B_CmpSensorFltLimtFlag) -> [xTmComprCtrl_B_CmpSensorFltLimtFlag]
  [sTmSigProces_Pw_i16ReqPwrForHeat] -> TAmbLimit/1(sTmSigProces_Pw_i16ReqPwrForHeat)
  [sTmSigProces_Te_s32TAmb] -> ?
  [rTmComprCtrl_n_u16CompRpmReqBoundary] -> TAmbLimit/2(rTmComprCtrl_n_u16CompRpmReqBoundary)
  [sTmRefriModeMgr_D_u8HPCurMode] -> ?
  TAmbLimit/1(rTmComprCtrl_n_u16CompMaxRpmTAmb) -> [rTmComprCtrl_n_u16CompMaxRpmTAmb]
  TAmbLimit/2(xTmComprCtrl_B_CmpAmbLimtFlag) -> [xTmComprCtrl_B_CmpAmbLimtFlag]

== system ScriptDemo/Create/Model/createModGotoAll/Before ==
  AFFaultLimit : Subsystem
  LoSidePFltLimt : Subsystem
  SensFaultLimit : Subsystem
  TAmbLimit : Subsystem
